simulink model "mpc_tgt_calc"  (R2022b)
settings: Solver=FixedStepDiscrete  StartTime=0.0  StopTime=2600  FixedStep=0.1  RelTol=1e-3
undefined symbols (not defined in the file): accl, alpha, alpha2, ang, beta, cnt_delay_accl_ratio, cnt_delay_decel_ratio, delay_accl, delay_v, dist, dt, ff_duty_front, ff_duty_l, ff_duty_r, ff_duty_roll, ff_duty_rpm_l, ff_duty_rpm_r, ideal_point, img_ang, img_dist, kanayama_point, pivot_state, sla_param, slip, slip_point, state, trj_diff, v, vx, vy, w
libraries: simulink_extras x1
(part 1 of 2)
settings Model: Creator=nao12  LastModifiedBy=naoto
settings SolverCC: AlgebraicLoopSolver=TrustRegion
settings DataIOCC: SaveOutput=off  SignalLogging=off  DSMLogging=off  SaveTime=off  ReturnWorkspaceOutputs=off
settings OptimizationCC: StrengthReduction=on  PassReuseOutputArgsAs=Individual arguments  ZeroExternalMemoryAtStartup=off  ZeroInternalMemoryAtStartup=off  OptimizeBlockOrder=speed  OptimizationPriority=Speed  OptimizationCustomize=off  MultiThreadedLoops=on  EfficientTunableParamExpr=on
settings DebuggingCC: ParameterTunabilityLossMsg=error  UnconnectedInputMsg=warning  UnconnectedOutputMsg=warning  UnconnectedLineMsg=warning  SFMachineParentedDataDiag=warning  ArithmeticOperatorsInVariantConditions=warning
settings ModelReferenceCC: EnableRefExpFcnMdlSchedulingChecks=on
settings SFSimCC: SimCustomHeaderCode="#include \"bus.h\""  SimUserIncludeDirs=../include/  MATLABDynamicMemAlloc=off  CustomCodeUndefinedFunction=UseInterfaceOnly  SimTargetLang=C++
settings RTWCC: Description=Embedded Coder  SystemTargetFile=ert.tlc  GenCodeOnly=on  TemplateMakefile=ert_default_tmf  GenerateReport=on  RTWUseSimCustomCode=on  CustomHeaderCode="#include \"bus.h\""  CustomInclude=../include/  Toolchain=GNU gcc/g++ | gmake (64-bit Linux)  IncludeHyperlinkInReport=on  LaunchReport=on  TargetLang=C++  GenerateTraceInfo=on  GenerateTraceReport=on  GenerateTraceReportSl=on  GenerateTraceReportSf=on  GenerateTraceReportEml=on  GenerateCodeMetricsReport=on  DLArmComputeVersion=19.05
settings CodeAppCC: GenerateComments=off  IgnoreCustomStorageClasses=off  OperatorAnnotations=on  SimulinkDataObjDesc=on  SFDataObjDesc=on  SimulinkBlockComments=off
settings ERTTargetCC: TargetLangStandard=C++11 (ISO)  GenerateSampleERTMain=on  SupportAbsoluteTime=off  CodeInterfacePackaging=C++ class  SupportComplex=off  ParenthesesLevel=Minimum  RootIOFormat=Structure reference  ERTCustomFileTemplate=example_file_process.tlc

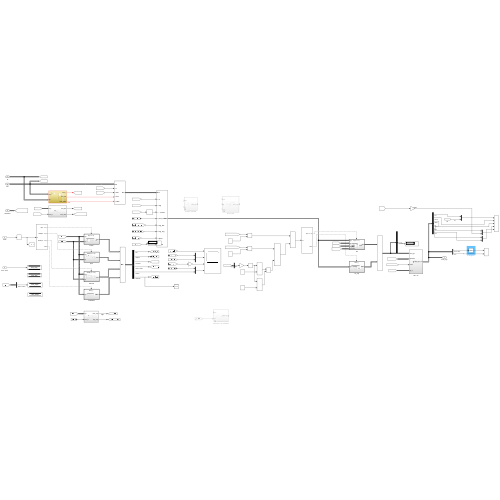
[thumbnail: Simulink's stored preview of the top-level diagram]
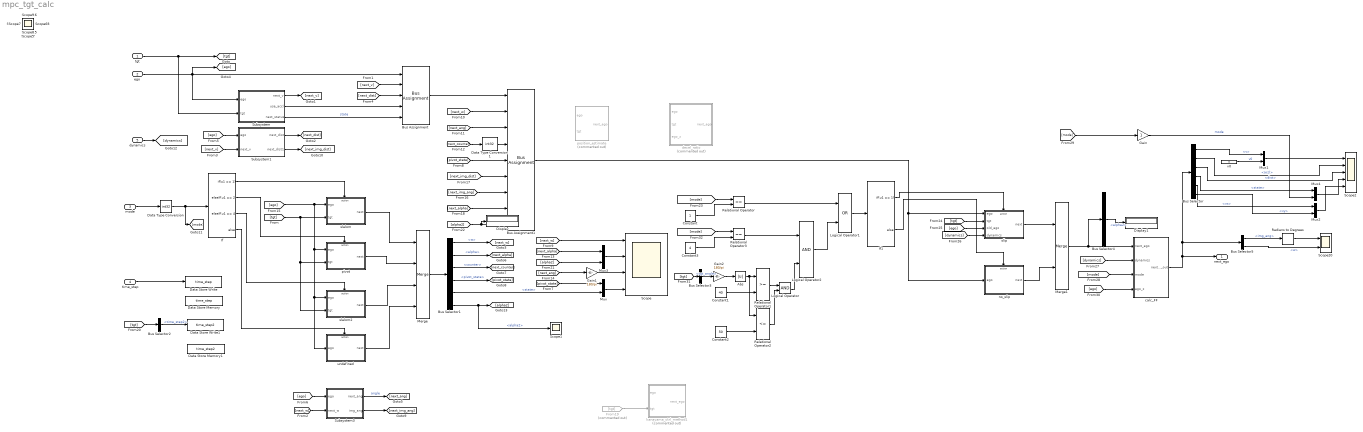
== system mpc_tgt_calc ==
  tgt : Inport  OutDataTypeStr=Bus: t_tgt  BusOutputAsStruct=on
  ego : Inport  Port=2  OutDataTypeStr=Bus: t_ego  BusOutputAsStruct=on
  mode : Inport  Port=3  OutDataTypeStr=int32
  time_step : Inport  Port=4  OutDataTypeStr=int32
  dynamics : Inport  Port=5  OutDataTypeStr=Bus: t_dynamics  BusOutputAsStruct=on
  Abs : Abs  SaturateOnIntegerOverflow=off
  Bus Assignment : BusAssignment  AssignedSignals=v,dist,accl,state
  Bus Assignment1 : BusAssignment  AssignedSignals=w,ang,sla_param.counter,pivot_state,img_dist,img_ang,alpha,alpha2
  Bus Selector : BusSelector  OutputSignals=v,accl,dist,state,slip.vx,slip.vy
  Bus Selector1 : BusSelector  OutputSignals=w,alpha,sla_param.counter,pivot_state,sla_param.state,alpha2
  Bus Selector2 : BusSelector  OutputSignals=time_step2
  Bus Selector3 : BusSelector  OutputSignals=tgt_angle
  Bus Selector4 : BusSelector  OutputSignals=alpha2
  Bus Selector5 : BusSelector  OutputSignals=img_ang,w
  Constant : Constant  OutDataTypeStr=int32
  Constant1 : Constant  Value=40  OutDataTypeStr=int32
  Constant2 : Constant  Value=50  OutDataTypeStr=int32
  Constant3 : Constant  Value=4  OutDataTypeStr=int32
  Data Store Memory : DataStoreMemory  DataStoreName=time_step  ReadBeforeWriteMsg=warning  WriteAfterWriteMsg=warning  WriteAfterReadMsg=warning  ShowAdditionalParam=off
  Data Store Memory1 : DataStoreMemory  DataStoreName=time_step2  ReadBeforeWriteMsg=warning  WriteAfterWriteMsg=warning  WriteAfterReadMsg=warning  ShowAdditionalParam=off
  Data Store Write : DataStoreWrite  DataStoreName=time_step  IndexOptions=Index vector (dialog)  Indices=1  OutputSizes=1
  Data Store Write1 : DataStoreWrite  DataStoreName=time_step2  IndexOptions=Index vector (dialog)  Indices=1  OutputSizes=1
  Data Type Conversion : DataTypeConversion  OutDataTypeStr=int32  SaturateOnIntegerOverflow=off  RndMeth=Floor
  Data Type Conversion1 : DataTypeConversion  OutDataTypeStr=int32  SaturateOnIntegerOverflow=off  RndMeth=Floor
  Display : Display
  Display1 : Display
  From19 : From  Commented=on  GotoTag=tgt
  Gain : Gain  OutDataTypeStr=int32
  Gain1 : Gain  Gain=180/pi
  Gain2 : Gain  Gain=180/pi
  If : If  IfExpression=u1 == 1  ElseIfExpressions=u1 == 2, u1 == 4
  If1 : If  IfExpression=u1 == 1
  Logical Operator : Logic  AllPortsSameDT=off  OutDataTypeStr=boolean
  Logical Operator1 : Logic  Operator=OR  AllPortsSameDT=off  OutDataTypeStr=boolean
  Logical Operator2 : Logic  AllPortsSameDT=off  OutDataTypeStr=boolean
  Merge : Merge  Inputs=4
  Merge1 : Merge
  Mux{,1..4} (5 alike) : Mux  Inputs=2
  Radians to Degrees : simulink_extras/Transformations/Radians to Degrees
  Relational Operator : RelationalOperator  Operator===  OutDataTypeStr=boolean  RndMeth=Simplest  InputSameDT=off
  Relational Operator1 : RelationalOperator  OutDataTypeStr=boolean  RndMeth=Simplest  InputSameDT=off
  Relational Operator2 : RelationalOperator  Operator=<=  OutDataTypeStr=boolean  RndMeth=Simplest  InputSameDT=off
  Relational Operator3 : RelationalOperator  Operator===  OutDataTypeStr=boolean  RndMeth=Simplest  InputSameDT=off
  Scope : Scope  NumInputPorts=4
  Scope{1,3..19} (18 alike) : Scope
  Scope2 : Scope  NumInputPorts=5
  Scope20 : Scope  NumInputPorts=2
  Subsystem : Subsystem
  Subsystem1 : Subsystem
  Subsystem3 : Subsystem
  calc_FF : Subsystem
  decel_ratio : Subsystem  Commented=on
  kanayama_ctrl_method1 : Subsystem  Commented=on
  no_slip : Subsystem  TreatAsAtomicUnit=on
  pivot : Subsystem  TreatAsAtomicUnit=on
  position_estimate : Subsystem  Commented=on
  slalom : Subsystem  TreatAsAtomicUnit=on
  slalom2 : Subsystem  TreatAsAtomicUnit=on
  slip : Subsystem  TreatAsAtomicUnit=on
  undefined : Subsystem  TreatAsAtomicUnit=on
  v0 : Constant  Value=0  OutDataTypeStr=single
  next_ego : Outport  OutDataTypeStr=Bus: t_ego
  wires:
  mode/1 -> Data Type Conversion/1
  tgt/1 -> [tgt], Subsystem/2(tgt)
  ego/1 -> Subsystem/1(ego), Bus Assignment/1, [ego]
  Data Type Conversion/1 -> [mode], If/1
  If/1 -> slalom/Action
  [tgt] -> slalom2/2(tgt), pivot/2(tgt), slalom/2(tgt)
  Bus Assignment/1 -> Bus Assignment1/1
  [next_v] -> Bus Assignment/2
  [next_dist] -> Bus Assignment/3
  Subsystem/1(next_v) -> [next_v]
  [next_v] -> Subsystem1/2(next_v)
  Subsystem1/1(next_dist) -> [next_dist]
  Subsystem/2(use_accl) -> Bus Assignment/4
  Subsystem/3(next_status) -> Bus Assignment/5  "state"
  [next_w] -> Subsystem3/2(next_w)
  [ego] -> Subsystem1/1(ego)
  [ego] -> Subsystem3/1(ego)
  Subsystem3/1(next_ang) -> [next_ang]  "angle"
  Bus Selector/4 -> Mux4/1  "<state>"
  Bus Selector/3 -> Scope2/3  "<dist>"
  [next_w] -> Bus Assignment1/2
  [next_ang] -> Bus Assignment1/3
  [next_counter] -> Data Type Conversion1/1
  Data Type Conversion1/1 -> Bus Assignment1/4
  [next_w] -> Scope/1
  [next_ang] -> Gain1/1
  If/2 -> pivot/Action
  [ego] -> slalom2/1(ego), undefined/1(ego), pivot/1(ego), slalom/1(ego)
  If/4 -> undefined/Action
  Merge/1 -> Bus Selector1/1
  Bus Selector1/1 -> [next_w]  "<w>"
  Bus Selector1/2 -> [next_alpha]  "<alpha>"
  Bus Selector1/3 -> [next_counter]  "<counter>"
  slalom/1(next) -> Merge/1
  pivot/1(next) -> Merge/2
  undefined/1(next) -> Merge/4
  Bus Selector1/4 -> [pivot_state]  "<pivot_state>"
  [pivot_state] -> Bus Assignment1/5
  Mux/1 -> Scope/4
  [pivot_state] -> Mux/1
  Bus Selector1/5 -> Mux/2  "<state>"
  Subsystem3/2(img_ang) -> [next_img_ang]
  [next_img_ang] -> Bus Assignment1/7
  Subsystem1/2(next_dist1) -> [next_img_dist]
  [next_img_dist] -> Bus Assignment1/6
  [next_alpha] -> Bus Assignment1/8
  From19/1 -> kanayama_ctrl_method1/2(tgt)
  time_step/1 -> Data Store Write/1
  slalom2/1(next) -> Merge/3
  If/3 -> slalom2/Action
  Bus Assignment1/1 -> no_slip/1(ego), slip/1(ego)
  If1/1 -> slip/Action
  slip/1(next) -> Merge1/1
  no_slip/1(next) -> Merge1/2
  If1/2 -> no_slip/Action
  Merge1/1 -> Bus Selector4/1, calc_FF/1(next_ego)
  [tgt] -> slip/2(tgt)
  [ego] -> slip/3(old_ego)
  Mux1/1 -> Scope2/1
  Bus Selector/1 -> Mux1/1  "<v>"
  v0/1 -> Mux1/2  "v0"
  [dynamics] -> calc_FF/2(dynamics)
  dynamics/1 -> [dynamics]
  [dynamics] -> slip/4(dynamics)
  Bus Selector2/1 -> Data Store Write1/1  "<time_step2>"
  [tgt] -> Bus Selector2/1
  Bus Selector1/6 -> Scope1/1, [alpha2]  "<alpha2>"
  Mux3/1 -> Scope/2
  [next_alpha] -> Mux3/1
  [alpha2] -> Mux3/2
  [alpha2] -> Display/1, Bus Assignment1/9
  calc_FF/1(next_ego_out) -> Bus Selector5/1, Bus Selector/1, next_ego/1
  [mode] -> calc_FF/3(mode)
  [mode] -> Gain/1
  Mux4/1 -> Scope2/4
  Gain/1 -> Mux4/2  "mode"
  Bus Selector/2 -> Scope2/2  "<accl>"
  Bus Selector/5 -> Mux2/1  "<vx>"
  Bus Selector/6 -> Mux2/2  "<vy>"
  Mux2/1 -> Scope2/5
  [ego] -> calc_FF/4(ego_z)
  Gain1/1 -> Scope/3
  [tgt] -> Bus Selector3/1
  Gain2/1 -> Abs/1
  [mode] -> Relational Operator/1
  Bus Selector3/1 -> Gain2/1  "<tgt_angle>"
  Relational Operator/1 -> Logical Operator1/1
  Constant/1 -> Relational Operator/2
  Abs/1 -> Relational Operator2/1, Relational Operator1/1
  Constant1/1 -> Relational Operator1/2
  Constant2/1 -> Relational Operator2/2
  Relational Operator1/1 -> Logical Operator/1
  Relational Operator2/1 -> Logical Operator/2
  Logical Operator1/1 -> If1/1
  [mode] -> Relational Operator3/1
  Relational Operator3/1 -> Logical Operator2/1
  Constant3/1 -> Relational Operator3/2
  Logical Operator/1 -> Logical Operator2/2
  Logical Operator2/1 -> Logical Operator1/2
  Bus Selector4/1 -> Display1/1  "<alpha2>"
  Bus Selector5/1 -> Radians to Degrees/1  "<img_ang>"
  Bus Selector5/2 -> Scope20/2  "<w>"
  Radians to Degrees/1 -> Scope20/1

== system mpc_tgt_calc/Subsystem ==
  ego : Inport
  tgt : Inport  Port=2
  Bus Selector2 : BusSelector  OutputSignals=v_max
  If : If  IfExpression=u1 >= 0
  Merge : Merge
  Merge1 : Merge
  Merge2 : Merge
  straight_ahead : Subsystem  TreatAsAtomicUnit=on
  straight_back : Subsystem  TreatAsAtomicUnit=on
  next_v : Outport
  use_accl : Outport  Port=2
  next_status : Outport  Port=3
  wires:
  tgt/1 -> [tgt], Bus Selector2/1
  Bus Selector2/1 -> If/1  "<v_max>"
  If/1 -> straight_ahead/Action
  ego/1 -> [ego]
  [ego] -> straight_ahead/1(ego)
  [tgt] -> straight_ahead/2(tgt)
  [ego] -> straight_back/1(ego)
  [tgt] -> straight_back/2(tgt)
  If/2 -> straight_back/Action
  straight_ahead/1(next_v) -> Merge/1
  straight_ahead/2(use_accl) -> Merge1/1
  straight_ahead/3(next_status) -> Merge2/1
  straight_back/1(next_v) -> Merge/2
  straight_back/2(use_accl) -> Merge1/2
  straight_back/3(next_status) -> Merge2/2
  Merge/1 -> next_v/1
  Merge1/1 -> use_accl/1
  Merge2/1 -> next_status/1

== system mpc_tgt_calc/Subsystem1 ==
  ego : Inport
  next_v : Inport  Port=2
  Add1 : Sum
  Add2 : Sum
  Bus Selector : BusSelector  OutputSignals=dist,img_dist
  Data Store Read : DataStoreRead  DataStoreName=time_step  IndexOptions=Index vector (dialog)  Indices=1  OutputSizes=1
  Data Type Conversion1 : DataTypeConversion  OutDataTypeStr=single  SaturateOnIntegerOverflow=off  RndMeth=Floor
  Data Type Conversion2 : DataTypeConversion  OutDataTypeStr=single  SaturateOnIntegerOverflow=off  RndMeth=Floor
  Data Type Conversion3 : DataTypeConversion  OutDataTypeStr=single  SaturateOnIntegerOverflow=off  RndMeth=Floor
  Gain1 : Gain  Gain=dt
  Product : Product
  next_dist : Outport
  next_dist1 : Outport  Port=2
  wires:
  ego/1 -> Bus Selector/1
  Bus Selector/1 -> Add1/1  "<dist>"
  Add1/1 -> Data Type Conversion1/1
  Data Type Conversion1/1 -> next_dist/1
  Add2/1 -> Data Type Conversion2/1
  Gain1/1 -> Add2/2, Add1/2
  Data Type Conversion2/1 -> next_dist1/1
  Bus Selector/2 -> Add2/1  "<img_dist>"
  Product/1 -> Gain1/1
  next_v/1 -> Product/1
  Data Store Read/1 -> Data Type Conversion3/1
  Data Type Conversion3/1 -> Product/2

== system mpc_tgt_calc/Subsystem3 ==
  ego : Inport
  next_w : Inport  Port=2
  Add1 : Sum
  Add2 : Sum
  Bus Selector : BusSelector  OutputSignals=ang,img_ang
  Data Store Read : DataStoreRead  DataStoreName=time_step  IndexOptions=Index vector (dialog)  Indices=1  OutputSizes=1
  Data Type Conversion1 : DataTypeConversion  OutDataTypeStr=single  SaturateOnIntegerOverflow=off  RndMeth=Floor
  Data Type Conversion2 : DataTypeConversion  OutDataTypeStr=single  SaturateOnIntegerOverflow=off  RndMeth=Floor
  Data Type Conversion3 : DataTypeConversion  OutDataTypeStr=single  SaturateOnIntegerOverflow=off  RndMeth=Floor
  Gain1 : Gain  Gain=dt
  Product : Product
  next_ang : Outport
  img_ang : Outport  Port=2
  wires:
  ego/1 -> Bus Selector/1
  Add1/1 -> Data Type Conversion1/1
  Bus Selector/1 -> Add1/1  "<ang>"
  Data Type Conversion1/1 -> next_ang/1
  Bus Selector/2 -> Add2/1  "<img_ang>"
  Data Type Conversion2/1 -> img_ang/1
  Add2/1 -> Data Type Conversion2/1
  Gain1/1 -> Add1/2, Add2/2
  Data Store Read/1 -> Data Type Conversion3/1
  Product/1 -> Gain1/1
  next_w/1 -> Product/1
  Data Type Conversion3/1 -> Product/2

== system mpc_tgt_calc/calc_FF ==
  next_ego : Inport
  dynamics : Inport  Port=2
  mode : Inport  Port=3
  ego_z : Inport  Port=4
  Add : Sum  Inputs=+-+
  Add1 : Sum  Inputs=+++
  Bus Assignment : BusAssignment  AssignedSignals=ff_duty_front,ff_duty_l,ff_duty_r,ff_duty_roll,ff_duty_rpm_r,ff_duty_rpm_l
  Mux : Mux  Inputs=2
  Mux1 : Mux  Inputs=2
  Scope : Scope  NumInputPorts=4
  Scope1 : Scope
  Subsystem : Subsystem
  calc_FF_Front : Subsystem
  calc_FF_Roll : Subsystem
  calc_counter_volt : Subsystem
  validation : Subsystem
  next_ego_out : Outport
  wires:
  next_ego/1 -> validation/1(next_ego)
  Bus Assignment/1 -> next_ego_out/1
  dynamics/1 -> calc_FF_Front/2(dynamics), calc_FF_Roll/2(dynamics), calc_counter_volt/2(dynamics)
  calc_counter_volt/1(left) -> [rpm_l_volt], Mux/1, Add/3  "rpm_l_volt"
  calc_counter_volt/2(right) -> Add1/3, [rpm_r_volt], Mux/2  "rpm_r_volt"
  Mux/1 -> Scope/4
  calc_FF_Front/1(front_volt) -> Subsystem/2(front_volt)
  calc_FF_Roll/1(roll_volt) -> [roll_volt], Scope1/1, Add1/2, Add/2, Scope/3
  Add1/1 -> Mux1/2, Bus Assignment/4  "FF_Right"
  Mux1/1 -> Scope/1
  Add/1 -> Mux1/1, Bus Assignment/3  "FF_Left"
  mode/1 -> Subsystem/3(mode)
  Subsystem/1(ff_front) -> Scope/2, Add1/1, Add/1, Bus Assignment/2
  validation/1(next_ego_out) -> calc_FF_Front/1(next_ego), calc_FF_Roll/1(next_ego), calc_counter_volt/1(next_ego), Subsystem/1(next_ego), Bus Assignment/1
  ego_z/1 -> validation/2(ego_z)
  [roll_volt] -> Bus Assignment/5
  [rpm_r_volt] -> Bus Assignment/6
  [rpm_l_volt] -> Bus Assignment/7

== system mpc_tgt_calc/decel_ratio ==
  ego : Inport
  tgt : Inport  Port=2
  ego_z : Inport  Port=3
  Bus Assignment : BusAssignment  AssignedSignals=delay_v,delay_accl,cnt_delay_accl_ratio,cnt_delay_decel_ratio
  Bus Selector : BusSelector  OutputSignals=accl
  Bus Selector1 : BusSelector  OutputSignals=v
  Data Store Read : DataStoreRead  DataStoreName=time_step  IndexOptions=Index vector (dialog)  Indices=1  OutputSizes=1
  Gain : Gain  Gain=dt
  If : If  ElseIfExpressions=u1 < 0
  If Action Subsystem : Subsystem  TreatAsAtomicUnit=on
  If Action Subsystem1 : Subsystem  TreatAsAtomicUnit=on
  If Action Subsystem2 : Subsystem  TreatAsAtomicUnit=on
  Merge : Merge  Inputs=3
  Merge1 : Merge  Inputs=3
  Merge2 : Merge  Inputs=3
  Product : Product
  next_ego : Outport
  wires:
  Bus Assignment/1 -> next_ego/1
  If/1 -> If Action Subsystem/Action
  ego/1 -> [ego], Bus Selector/1, Bus Assignment/1
  [ego] -> If Action Subsystem/1(ego)
  Bus Selector/1 -> If/1  "<accl>"
  tgt/1 -> If Action Subsystem/2(tgt), If Action Subsystem1/2(tgt)
  If/2 -> If Action Subsystem1/Action
  If/3 -> If Action Subsystem2/Action
  [ego] -> If Action Subsystem1/1(ego)
  If Action Subsystem/1(ff_accl) -> Merge/1
  If Action Subsystem1/1(ff_accl) -> Merge/2
  If Action Subsystem2/1(ff_accl) -> Merge/3
  If Action Subsystem/2(cnt_delay_accl_ratio) -> Merge1/1
  If Action Subsystem1/2(cnt_delay_accl_ratio) -> Merge1/2
  If Action Subsystem2/2(cnt_delay_accl_ratio) -> Merge1/3
  If Action Subsystem/3(cnt_delay_decel_ratio) -> Merge2/1
  If Action Subsystem1/3(cnt_delay_decel_ratio) -> Merge2/2
  If Action Subsystem2/3(cnt_delay_decel_ratio) -> Merge2/3
  Merge/1 -> Bus Assignment/3
  Merge1/1 -> Bus Assignment/4
  Merge2/1 -> Bus Assignment/5
  [ego] -> If Action Subsystem2/1(ego)
  ego_z/1 -> Bus Selector1/1
  Data Store Read/1 -> Product/1
  Gain/1 -> Product/2
  Bus Selector1/1 -> Gain/1  "<v>"
  Product/1 -> Bus Assignment/2

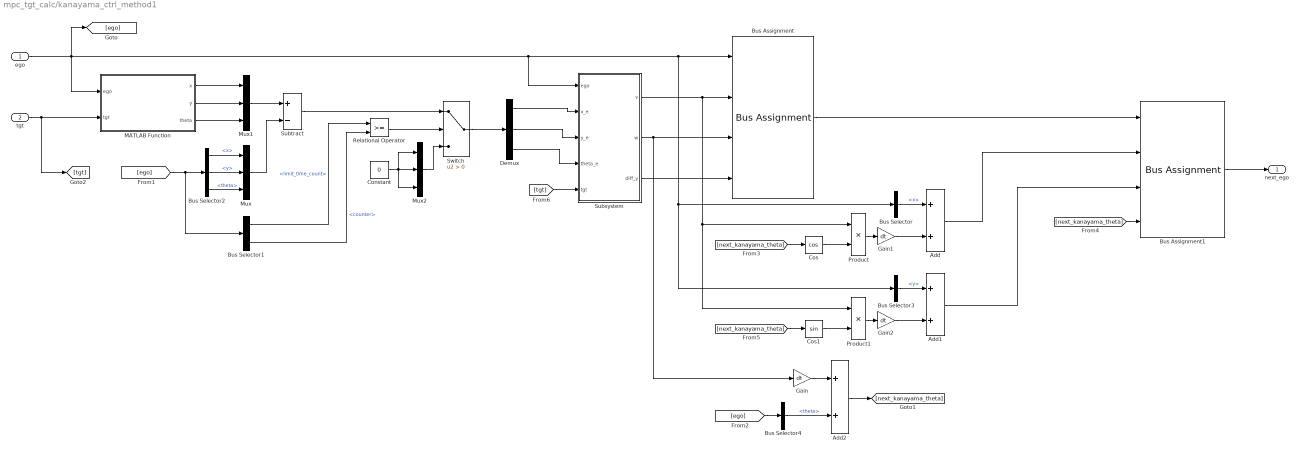
== system mpc_tgt_calc/kanayama_ctrl_method1 ==
  ego : Inport
  tgt : Inport  Port=2
  Add : Sum
  Add1 : Sum
  Add2 : Sum
  Bus Assignment : BusAssignment  AssignedSignals=kanayama_point.v,kanayama_point.w,kanayama_point.y
  Bus Assignment1 : BusAssignment  AssignedSignals=kanayama_point.x,kanayama_point.y,kanayama_point.theta
  Bus Selector : BusSelector  OutputSignals=kanayama_point.x
  Bus Selector1 : BusSelector  OutputSignals=sla_param.limit_time_count,sla_param.counter
  Bus Selector2 : BusSelector  OutputSignals=slip_point.x,slip_point.y,slip_point.theta
  Bus Selector3 : BusSelector  OutputSignals=kanayama_point.y
  Bus Selector4 : BusSelector  OutputSignals=kanayama_point.theta
  Constant : Constant  Value=0  OutDataTypeStr=single
  Cos : Trigonometry  Operator=cos
  Cos1 : Trigonometry
  Demux : Demux  Outputs=3
  Gain : Gain  Gain=dt
  Gain1 : Gain  Gain=dt
  Gain2 : Gain  Gain=dt
  MATLAB Function : MATLAB Function  TreatAsAtomicUnit=on
  Mux : Mux  Inputs=3
  Mux1 : Mux  Inputs=3
  Mux2 : Mux  Inputs=3
  Product : Product
  Product1 : Product
  Relational Operator : RelationalOperator  OutDataTypeStr=boolean  RndMeth=Simplest  InputSameDT=off
  Subsystem : Subsystem
  Subtract : Sum  Inputs=+-
  Switch : Switch  Criteria=u2 > Threshold  SaturateOnIntegerOverflow=off  InputSameDT=off
  next_ego : Outport
  wires:
  tgt/1 -> [tgt], MATLAB Function/2(tgt)
  Bus Selector2/1 -> Mux/1  "<x>"
  Bus Selector2/2 -> Mux/2  "<y>"
  Bus Selector2/3 -> Mux/3  "<theta>"
  MATLAB Function/1(x) -> Mux1/1
  MATLAB Function/2(y) -> Mux1/2
  MATLAB Function/3(theta) -> Mux1/3
  Mux1/1 -> Subtract/1
  Mux/1 -> Subtract/2
  Switch/1 -> Demux/1
  Bus Selector1/1 -> Relational Operator/1  "<limit_time_count>"
  Bus Selector1/2 -> Relational Operator/2  "<counter>"
  Relational Operator/1 -> Switch/2
  Subtract/1 -> Switch/1
  Mux2/1 -> Switch/3
  Constant/1 -> Mux2/1, Mux2/2, Mux2/3
  Bus Assignment/1 -> Bus Assignment1/1
  Demux/1 -> Subsystem/2(x_e)
  Demux/2 -> Subsystem/3(y_e)
  Demux/3 -> Subsystem/4(theta_e)
  Subsystem/2(w) -> Gain/1, Bus Assignment/3
  Product/1 -> Gain1/1
  Bus Selector/1 -> Add/1  "<x>"
  Add/1 -> Bus Assignment1/2
  Add1/1 -> Bus Assignment1/3
  Cos/1 -> Product/2
  Subsystem/1(v) -> Product/1, Product1/1, Bus Assignment/2
  [next_kanayama_theta] -> Cos/1
  Gain1/1 -> Add/2
  Cos1/1 -> Product1/2
  Gain2/1 -> Add1/2
  ego/1 -> MATLAB Function/1(ego), [ego], Subsystem/1(ego), Bus Selector3/1, Bus Selector/1, Bus Assignment/1
  Product1/1 -> Gain2/1
  Bus Assignment1/1 -> next_ego/1
  [ego] -> Bus Selector1/1, Bus Selector2/1
  [ego] -> Bus Selector4/1
  Gain/1 -> Add2/1
  Bus Selector4/1 -> Add2/2  "<theta>"
  Add2/1 -> [next_kanayama_theta]
  Bus Selector3/1 -> Add1/1  "<y>"
  [next_kanayama_theta] -> Bus Assignment1/4
  [next_kanayama_theta] -> Cos1/1
  [tgt] -> Subsystem/5(tgt)
  Subsystem/3(diff_y) -> Bus Assignment/4

== system mpc_tgt_calc/no_slip ==
  ego : Inport
  Action Port : ActionPort  ActionPortLabel=else
  Bus Assignment : BusAssignment  AssignedSignals=beta,vx,vy,v
  Bus Assignment1 : BusAssignment  AssignedSignals=slip
  Bus Selector : BusSelector  OutputSignals=slip,v
  Constant : Constant  Value=0  OutDataTypeStr=single
  Gain : Gain  Gain=0.001
  Gain1 : Gain  Gain=0.001
  next : Outport
  wires:
  Bus Assignment1/1 -> next/1
  Bus Selector/1 -> Bus Assignment/1  "<slip>"
  ego/1 -> Bus Selector/1, Bus Assignment1/1
  Bus Assignment/1 -> Bus Assignment1/2
  Constant/1 -> Bus Assignment/4, Bus Assignment/2
  Bus Selector/2 -> Gain/1, Gain1/1  "<v>"
  Gain/1 -> Bus Assignment/5
  Gain1/1 -> Bus Assignment/3

== system mpc_tgt_calc/pivot ==
  ego : Inport
  tgt : Inport  Port=2
  Action Port : ActionPort  ActionPortLabel=elseif(u1 == 2)
  Abs : Abs  SaturateOnIntegerOverflow=off
  Abs1 : Abs  SaturateOnIntegerOverflow=off
  Add : Sum
  Bus Assignment : BusAssignment  AssignedSignals=w,alpha,alpha2,pivot_state
  Bus Assignment1 : BusAssignment  AssignedSignals=w,alpha,alpha2,pivot_state
  Bus Selector : BusSelector  OutputSignals=w
  Bus Selector1 : BusSelector  OutputSignals=ang
  Bus Selector2 : BusSelector  OutputSignals=tgt_angle
  Constant : Constant  Value=0  OutDataTypeStr=single
  Constant1 : Constant  Value=3  OutDataTypeStr=int32
  Data Store Read : DataStoreRead  DataStoreName=time_step  IndexOptions=Index vector (dialog)  Indices=1  OutputSizes=1
  Data Type Conversion1 : DataTypeConversion  OutDataTypeStr=single  SaturateOnIntegerOverflow=off  RndMeth=Floor
  Data Type Conversion2 : DataTypeConversion  OutDataTypeStr=single  SaturateOnIntegerOverflow=off  RndMeth=Floor
  Data Type Conversion3 : DataTypeConversion  OutDataTypeStr=single  SaturateOnIntegerOverflow=off  RndMeth=Floor
  Gain : Gain  Gain=dt
  Product : Product
  Relational Operator1 : RelationalOperator  Operator=<  OutDataTypeStr=boolean  RndMeth=Simplest  InputSameDT=off
  Subsystem : Subsystem
  Switch2 : Switch  Criteria=u2 > Threshold  SaturateOnIntegerOverflow=off  InputSameDT=off
  next : Outport
  wires:
  ego/1 -> Subsystem/1(ego), Bus Selector/1, Bus Assignment/1, [ego]
  Subsystem/1(next_alpha) -> Data Type Conversion1/1, Gain/1
  Bus Selector/1 -> Add/1  "<w>"
  Add/1 -> Data Type Conversion2/1
  Data Type Conversion2/1 -> Bus Assignment/2
  tgt/1 -> [tgt], Subsystem/2(tgt)
  Data Type Conversion1/1 -> Bus Assignment/4, Bus Assignment/3
  Subsystem/2(state_out) -> Bus Assignment/5
  Bus Assignment/1 -> Bus Assignment1/1, Switch2/1
  Relational Operator1/1 -> Switch2/2
  Bus Selector2/1 -> Abs1/1  "<tgt_angle>"
  Abs/1 -> Relational Operator1/1
  [ego] -> Bus Selector1/1
  [tgt] -> Bus Selector2/1
  Bus Selector1/1 -> Abs/1  "<ang>"
  Abs1/1 -> Relational Operator1/2
  Switch2/1 -> next/1
  Constant/1 -> Bus Assignment1/4, Bus Assignment1/3, Bus Assignment1/2
  Constant1/1 -> Bus Assignment1/5
  Bus Assignment1/1 -> Switch2/3
  Data Store Read/1 -> Data Type Conversion3/1
  Gain/1 -> Product/1
  Product/1 -> Add/2
  Data Type Conversion3/1 -> Product/2

== system mpc_tgt_calc/position_estimate ==
  ego : Inport
  tgt : Inport  Port=2
  Add : Sum
  Add1 : Sum
  Bus Assignment : BusAssignment  AssignedSignals=ideal_point.x,ideal_point.y,ideal_point.theta
  Bus Assignment1 : BusAssignment  AssignedSignals=trj_diff.x,trj_diff.y,trj_diff.theta
  Bus Selector : BusSelector  OutputSignals=ideal_point.x,v,img_ang
  Bus Selector1 : BusSelector  OutputSignals=ideal_point.y,v,img_ang
  Bus Selector2 : BusSelector  OutputSignals=ideal_point.theta
  Bus Selector3 : BusSelector  OutputSignals=ideal_point.x,ideal_point.y
  Bus Selector4 : BusSelector  OutputSignals=slip_point.x,slip_point.y
  Bus Selector5 : BusSelector  OutputSignals=img_ang,slip_point.theta
  Cos : Trigonometry  Operator=cos
  Cos1 : Trigonometry
  Data Store Read1 : DataStoreRead  DataStoreName=time_step  IndexOptions=Index vector (dialog)  Indices=1  OutputSizes=1
  Gain1 : Gain  Gain=dt
  Gain2 : Gain  Gain=dt
  Gain5 : Gain
  Gain6 : Gain
  Mux : Mux  Inputs=2
  Mux1 : Mux  Inputs=2
  Product{,1..3} (4 alike) : Product
  Scope : Scope  NumInputPorts=2
  Subtract : Sum  Inputs=+-
  Subtract1 : Sum  Inputs=+-
  Subtract2 : Sum  Inputs=+-
  slipped_position_estimate : Subsystem
  next_ego : Outport
  wires:
  ego/1 -> slipped_position_estimate/1(ego), Bus Selector1/1, Bus Selector2/1, Bus Selector/1
  Bus Selector/1 -> Add/1  "<x>"
  Bus Selector/2 -> Product/1  "<v>"
  Bus Selector/3 -> Cos/1  "<img_ang>"
  Cos/1 -> Product/2
  Product/1 -> Gain1/1
  Bus Selector1/2 -> Product1/1  "<v>"
  Bus Selector1/1 -> Add1/1  "<y>"
  Product1/1 -> Gain2/1
  Bus Selector1/3 -> Cos1/1  "<img_ang>"
  Cos1/1 -> Product1/2
  Bus Selector2/1 -> Bus Assignment/4  "<theta>"
  Add1/1 -> Bus Assignment/3
  Add/1 -> Bus Assignment/2
  Bus Selector3/1 -> Subtract/1  "<x>"
  Bus Selector3/2 -> Subtract1/1  "<y>"
  slipped_position_estimate/1(next_ego) -> Bus Assignment/1
  Bus Selector4/1 -> Subtract/2  "<x>"
  Bus Selector4/2 -> Subtract1/2  "<y>"
  Subtract/1 -> Bus Assignment1/2, Mux1/1  "slip_diff_x"
  Subtract1/1 -> Mux1/2, Bus Assignment1/3  "slip_diff_y"
  Bus Assignment/1 -> Bus Selector5/1, Bus Selector3/1, Bus Assignment1/1, Bus Selector4/1
  Bus Selector5/2 -> Gain6/1  "<theta>"
  Gain6/1 -> Mux/2, Subtract2/2  "slipped_angle"
  Gain5/1 -> Mux/1, Subtract2/1  "ideal_angle"
  Bus Selector5/1 -> Gain5/1  "<img_ang>"
  Mux/1 -> Scope/2
  Mux1/1 -> Scope/1
  Bus Assignment1/1 -> next_ego/1
  Subtract2/1 -> Bus Assignment1/4  "slip_diff_theta"
  tgt/1 -> slipped_position_estimate/2(tgt)
  Product2/1 -> Add/2
  Gain1/1 -> Product2/1
  Product3/1 -> Add1/2
  Data Store Read1/1 -> Product3/1, Product2/2
  Gain2/1 -> Product3/2

== system mpc_tgt_calc/slalom ==
  ego : Inport
  tgt : Inport  Port=2
  Action Port : ActionPort  ActionPortLabel=if(u1 == 1)
  Bus Assignment : BusAssignment  AssignedSignals=w,alpha,sla_param.counter,alpha2
  Data Type Conversion : DataTypeConversion  OutDataTypeStr=int32  SaturateOnIntegerOverflow=off  RndMeth=Floor
  Data Type Conversion1 : DataTypeConversion  OutDataTypeStr=single  SaturateOnIntegerOverflow=off  RndMeth=Floor
  Data Type Conversion2 : DataTypeConversion  OutDataTypeStr=single  SaturateOnIntegerOverflow=off  RndMeth=Floor
  Data Type Conversion3 : DataTypeConversion  OutDataTypeStr=single  SaturateOnIntegerOverflow=off  RndMeth=Floor
  Subsystem2 : Subsystem
  next : Outport
  wires:
  ego/1 -> Subsystem2/1(ego), Bus Assignment/1
  tgt/1 -> Subsystem2/2(tgt)
  Bus Assignment/1 -> next/1
  Subsystem2/1(next_w) -> Data Type Conversion1/1
  Subsystem2/2(next_alpha) -> Data Type Conversion2/1
  Subsystem2/3(next_count) -> Data Type Conversion/1
  Data Type Conversion/1 -> Bus Assignment/4
  Data Type Conversion1/1 -> Bus Assignment/2
  Data Type Conversion2/1 -> Bus Assignment/3
  Data Type Conversion3/1 -> Bus Assignment/5
  Subsystem2/4(next_alpha2) -> Data Type Conversion3/1

== system mpc_tgt_calc/slalom2 ==
  ego : Inport
  tgt : Inport  Port=2
  Action Port : ActionPort  ActionPortLabel=elseif( u1 == 4)
  Abs : Abs  SaturateOnIntegerOverflow=off
  Abs1 : Abs  SaturateOnIntegerOverflow=off
  Add : Sum
  Bus Assignment : BusAssignment  AssignedSignals=w,alpha,pivot_state
  Bus Assignment1 : BusAssignment  AssignedSignals=w,alpha,alpha2,pivot_state
  Bus Selector : BusSelector  OutputSignals=w
  Bus Selector1 : BusSelector  OutputSignals=img_ang
  Bus Selector2 : BusSelector  OutputSignals=tgt_angle
  Bus Selector3 : BusSelector  OutputSignals=w
  Constant : Constant  Value=0  OutDataTypeStr=single
  Constant1 : Constant  Value=3  OutDataTypeStr=int32
  Data Store Read : DataStoreRead  DataStoreName=time_step  IndexOptions=Index vector (dialog)  Indices=1  OutputSizes=1
  Data Store Read1 : DataStoreRead  DataStoreName=time_step  IndexOptions=Index vector (dialog)  Indices=1  OutputSizes=1
  Data Type Conversion{1..4} (4 alike) : DataTypeConversion  OutDataTypeStr=single  SaturateOnIntegerOverflow=off  RndMeth=Floor
  Divide : Product  Inputs=*/
  Gain : Gain  Gain=dt
  Gain1 : Gain  Gain=dt
  Product : Product
  Relational Operator1 : RelationalOperator  Operator=<  OutDataTypeStr=boolean  RndMeth=Simplest  InputSameDT=off
  Scope : Scope
  Subsystem : Subsystem
  Subtract : Sum  Inputs=+-
  Switch2 : Switch  Criteria=u2 > Threshold  SaturateOnIntegerOverflow=off  InputSameDT=off
  next : Outport
  wires:
  Subsystem/1(next_alpha) -> Data Type Conversion1/1, Gain/1
  Bus Selector/1 -> Add/1  "<w>"
  Add/1 -> Data Type Conversion2/1
  Data Type Conversion2/1 -> Bus Assignment/2
  Data Type Conversion1/1 -> Bus Assignment/3
  Subsystem/2(state_out) -> Bus Assignment/4
  Bus Assignment/1 -> Bus Assignment1/1, Switch2/1
  Relational Operator1/1 -> Switch2/2
  Bus Selector2/1 -> Abs1/1  "<tgt_angle>"
  Abs/1 -> Relational Operator1/1
  ego/1 -> Bus Selector3/1, Subsystem/1(ego), Bus Selector/1, Bus Selector1/1, Bus Assignment/1
  tgt/1 -> Bus Selector2/1, Subsystem/2(tgt)
  Bus Selector1/1 -> Abs/1  "<img_ang>"
  Abs1/1 -> Relational Operator1/2
  Switch2/1 -> next/1
  Constant1/1 -> Bus Assignment1/5
  Bus Assignment1/1 -> Switch2/3
  Data Store Read/1 -> Data Type Conversion3/1
  Gain/1 -> Product/1
  Product/1 -> Add/2
  Constant/1 -> Subtract/1, Bus Assignment1/4, Bus Assignment1/3, Bus Assignment1/2
  Bus Selector3/1 -> Subtract/2  "<w>"
  Subtract/1 -> Divide/1
  Data Store Read1/1 -> Data Type Conversion4/1
  Gain1/1 -> Divide/2
  Data Type Conversion3/1 -> Product/2
  Data Type Conversion4/1 -> Gain1/1

== system mpc_tgt_calc/slip ==
  ego : Inport
  tgt : Inport  Port=2
  old_ego : Inport  Port=3
  dynamics : Inport  Port=4
  Action Port : ActionPort  ActionPortLabel=if(u1 == 1)
  Bus Assignment1 : BusAssignment  AssignedSignals=slip,v,accl
  Bus Selector3 : BusSelector  OutputSignals=v
  Subsystem : Subsystem
  next : Outport
  wires:
  ego/1 -> Subsystem/1(next_ego), Bus Assignment1/1
  Bus Assignment1/1 -> next/1
  old_ego/1 -> Bus Selector3/1
  Subsystem/1(slip_param) -> Bus Assignment1/2
  tgt/1 -> Subsystem/2(tgt)
  Bus Selector3/1 -> Subsystem/3(old_v)  "<v>"
  Subsystem/2(v) -> Bus Assignment1/3
  Subsystem/3(accl) -> Bus Assignment1/4
  dynamics/1 -> Subsystem/4(dynamics)

== system mpc_tgt_calc/undefined ==
  ego : Inport
  Action Port : ActionPort  ActionPortLabel=else
  Bus Assignment1 : BusAssignment  AssignedSignals=w,alpha,alpha2
  Bus Selector3 : BusSelector  OutputSignals=w
  Constant : Constant  Value=0  OutDataTypeStr=single
  Data Store Read : DataStoreRead  DataStoreName=time_step  IndexOptions=Index vector (dialog)  Indices=1  OutputSizes=1
  Data Type Conversion1 : DataTypeConversion  OutDataTypeStr=single  SaturateOnIntegerOverflow=off  RndMeth=Floor
  Data Type Conversion2 : DataTypeConversion  OutDataTypeStr=single  SaturateOnIntegerOverflow=off  RndMeth=Floor
  Divide : Product  Inputs=*/
  Gain : Gain  Gain=dt
  Subtract : Sum  Inputs=+-
  next : Outport
  wires:
  ego/1 -> Bus Selector3/1, Bus Assignment1/1
  Gain/1 -> Divide/2
  Bus Selector3/1 -> Subtract/2  "<w>"
  Subtract/1 -> Divide/1
  Constant/1 -> Subtract/1, Bus Assignment1/2
  Divide/1 -> Bus Assignment1/4, Bus Assignment1/3
  Bus Assignment1/1 -> next/1
  Data Store Read/1 -> Data Type Conversion1/1
  Data Type Conversion1/1 -> Gain/1

== system mpc_tgt_calc/Subsystem/straight_ahead ==
  ego : Inport
  tgt : Inport  Port=2
  Action Port : ActionPort  ActionPortLabel=if(u1 >= 0)
  Add : Sum
  Bus Selector : BusSelector  OutputSignals=v
  Bus Selector1 : BusSelector  OutputSignals=v_max
  Constant : Constant  Value=0  OutDataTypeStr=single
  Data Store Read : DataStoreRead  DataStoreName=time_step  IndexOptions=Index vector (dialog)  Indices=1  OutputSizes=1
  Data Type Conversion1 : DataTypeConversion  OutDataTypeStr=single  SaturateOnIntegerOverflow=off  RndMeth=Floor
  Data Type Conversion2 : DataTypeConversion  OutDataTypeStr=single  SaturateOnIntegerOverflow=off  RndMeth=Floor
  Gain : Gain  Gain=dt
  Max : MinMax  Function=max  Inputs=2
  Min : MinMax  Inputs=2
  Product : Product
  Subsystem : Subsystem
  next_v : Outport
  use_accl : Outport  Port=2
  next_status : Outport  Port=3
  wires:
  Max/1 -> next_v/1
  Subsystem/1(use_accl) -> use_accl/1, Gain/1
  Constant/1 -> Max/2
  Bus Selector/1 -> Add/1  "<v>"
  ego/1 -> Subsystem/1(ego), Bus Selector/1
  tgt/1 -> Subsystem/2(tgt), Bus Selector1/1
  Data Type Conversion2/1 -> Min/2
  Min/1 -> Max/1  "velocity"
  Bus Selector1/1 -> Min/1  "<v_max>"
  Subsystem/2(next_state) -> next_status/1
  Add/1 -> Data Type Conversion2/1
  Data Store Read/1 -> Data Type Conversion1/1
  Product/1 -> Add/2
  Gain/1 -> Product/2
  Data Type Conversion1/1 -> Product/1

== system mpc_tgt_calc/Subsystem/straight_back ==
  ego : Inport
  tgt : Inport  Port=2
  Action Port : ActionPort  ActionPortLabel=else
  Add : Sum
  Bus Selector : BusSelector  OutputSignals=v
  Bus Selector1 : BusSelector  OutputSignals=v_max
  Constant : Constant  Value=0  OutDataTypeStr=single
  Data Store Read : DataStoreRead  DataStoreName=time_step  IndexOptions=Index vector (dialog)  Indices=1  OutputSizes=1
  Data Type Conversion1 : DataTypeConversion  OutDataTypeStr=single  SaturateOnIntegerOverflow=off  RndMeth=Floor
  Data Type Conversion2 : DataTypeConversion  OutDataTypeStr=single  SaturateOnIntegerOverflow=off  RndMeth=Floor
  Gain : Gain  Gain=dt
  Max : MinMax  Inputs=2
  Min : MinMax  Function=max  Inputs=2
  Product : Product
  Subsystem : Subsystem
  next_v : Outport
  use_accl : Outport  Port=2
  next_status : Outport  Port=3
  wires:
  Max/1 -> next_v/1
  Subsystem/1(use_accl) -> use_accl/1, Gain/1
  Constant/1 -> Max/2
  Bus Selector/1 -> Add/1  "<v>"
  ego/1 -> Subsystem/1(ego), Bus Selector/1
  tgt/1 -> Subsystem/2(tgt), Bus Selector1/1
  Data Type Conversion2/1 -> Min/2
  Min/1 -> Max/1  "velocity"
  Bus Selector1/1 -> Min/1  "<v_max>"
  Subsystem/2(next_state) -> next_status/1
  Add/1 -> Data Type Conversion2/1
  Data Store Read/1 -> Data Type Conversion1/1
  Product/1 -> Add/2
  Gain/1 -> Product/2
  Data Type Conversion1/1 -> Product/1

== system mpc_tgt_calc/calc_FF/Subsystem ==
  next_ego : Inport
  front_volt : Inport  Port=2
  mode : Inport  Port=3
  Bus Selector : BusSelector  OutputSignals=state
  If : If  NumInputs=2  IfExpression=(u2==0 | u2==3 ) & (u1==0)
  If Action Subsystem : Subsystem  TreatAsAtomicUnit=on
  If Action Subsystem1 : Subsystem  TreatAsAtomicUnit=on
  Merge : Merge
  ff_front : Outport
  wires:
  next_ego/1 -> If Action Subsystem/2(next_ego), Bus Selector/1
  Bus Selector/1 -> If/1  "<state>"
  mode/1 -> If/2
  If/1 -> If Action Subsystem/Action
  If/2 -> If Action Subsystem1/Action
  front_volt/1 -> If Action Subsystem1/1(front_volt), If Action Subsystem/1(front_volt)
  If Action Subsystem/1(Out1) -> Merge/1
  If Action Subsystem1/1(Out1) -> Merge/2
  Merge/1 -> ff_front/1

== system mpc_tgt_calc/calc_FF/calc_FF_Front ==
  next_ego : Inport
  dynamics : Inport  Port=2
  Bus Selector : BusSelector  OutputSignals=accl
  Bus Selector1 : BusSelector  OutputSignals=mass,tire,resist
  Bus Selector2 : BusSelector  OutputSignals=gear_ratio,km
  Divide : Product  Inputs=*/
  Gain1 : Gain  Gain=0.001
  Gain4 : Gain  Gain=0.001
  Product : Product  Inputs=4
  Product1 : Product
  front_volt : Outport
  wires:
  Bus Selector1/1 -> Product/2  "<mass>"
  dynamics/1 -> Bus Selector2/1, Bus Selector1/1
  next_ego/1 -> Bus Selector/1
  Bus Selector/1 -> Gain4/1  "<accl>"
  Gain4/1 -> Product/1
  Bus Selector1/2 -> Gain1/1  "<tire>"
  Bus Selector1/3 -> Product/4  "<resist>"
  Gain1/1 -> Product/3
  Bus Selector2/2 -> Product1/2  "<km>"
  Bus Selector2/1 -> Product1/1  "<gear_ratio>"
  Product/1 -> Divide/1
  Product1/1 -> Divide/2
  Divide/1 -> front_volt/1

== system mpc_tgt_calc/calc_FF/calc_FF_Roll ==
  next_ego : Inport
  dynamics : Inport  Port=2
  Bus Selector : BusSelector  OutputSignals=alpha2
  Bus Selector1 : BusSelector  OutputSignals=lm,tire,resist
  Bus Selector2 : BusSelector  OutputSignals=gear_ratio,km,tread
  Display{,1..5} (6 alike) : Display
  Divide : Product  Inputs=*/
  Divide1 : Product  Inputs=*/
  Gain1 : Gain  Gain=0.001
  Gain2 : Gain  Gain=0.001
  Product : Product  Inputs=4
  Product1 : Product
  Scope : Scope  NumInputPorts=2
  Scope2 : Scope
  roll_volt : Outport
  wires:
  Bus Selector1/3 -> Product/4, Display5/1  "<resist>"
  Bus Selector/1 -> Display3/1, Product/1  "<alpha2>"
  Bus Selector1/2 -> Gain1/1  "<tire>"
  next_ego/1 -> Bus Selector/1
  Bus Selector1/1 -> Display4/1, Product/2  "<lm>"
  dynamics/1 -> Bus Selector2/1, Bus Selector1/1
  Product1/1 -> Display2/1, Divide/2
  Gain1/1 -> Product/3
  Divide/1 -> Scope/1, Display/1, Divide1/1
  Product/1 -> Display1/1, Divide/1
  Bus Selector2/1 -> Product1/1  "<gear_ratio>"
  Bus Selector2/2 -> Product1/2  "<km>"
  Bus Selector2/3 -> Gain2/1  "<tread>"
  Gain2/1 -> Divide1/2, Scope2/1
  Divide1/1 -> roll_volt/1

== system mpc_tgt_calc/calc_FF/calc_counter_volt ==
  next_ego : Inport
  dynamics : Inport  Port=2
  Add : Sum  Inputs=+-
  Add1 : Sum
  Bus Selector : BusSelector  OutputSignals=v,w
  Bus Selector1 : BusSelector  OutputSignals=tread
  Bus Selector2 : BusSelector  OutputSignals=ke,tire
  Divide : Product  Inputs=*/
  Divide1 : Product  Inputs=*/
  Gain : Gain  Gain=0.5
  Gain1 : Gain  Gain=0.5
  Gain2 : Gain  Gain=30/pi
  Gain3 : Gain  Gain=30/pi
  Gain4 : Gain  Gain=0.001
  Gain5 : Gain  Gain=0.001
  Gain6 : Gain  Gain=0.001
  Product : Product
  Product1 : Product
  Product2 : Product
  left : Outport
  right : Outport  Port=2
  wires:
  next_ego/1 -> Bus Selector/1
  dynamics/1 -> Bus Selector2/1, Bus Selector1/1
  Bus Selector/1 -> Gain4/1  "<v>"
  Bus Selector/2 -> Product/1  "<w>"
  Bus Selector1/1 -> Gain5/1  "<tread>"
  Gain/1 -> Product/2
  Product/1 -> Add1/2, Add/2
  Add/1 -> Product1/1
  Add1/1 -> Product2/1
  Bus Selector2/1 -> [ke]  "<ke>"
  Bus Selector2/2 -> Gain6/1  "<tire>"
  Gain1/1 -> [tire_2]
  [ke] -> Product1/2
  Product1/1 -> Gain2/1
  [tire_2] -> Divide/2
  [tire_2] -> Divide1/2
  Gain2/1 -> Divide/1
  Product2/1 -> Gain3/1
  Gain3/1 -> Divide1/1
  [ke] -> Product2/2
  Divide/1 -> left/1
  Divide1/1 -> right/1
  Gain4/1 -> Add1/1, Add/1
  Gain5/1 -> Gain/1
  Gain6/1 -> Gain1/1

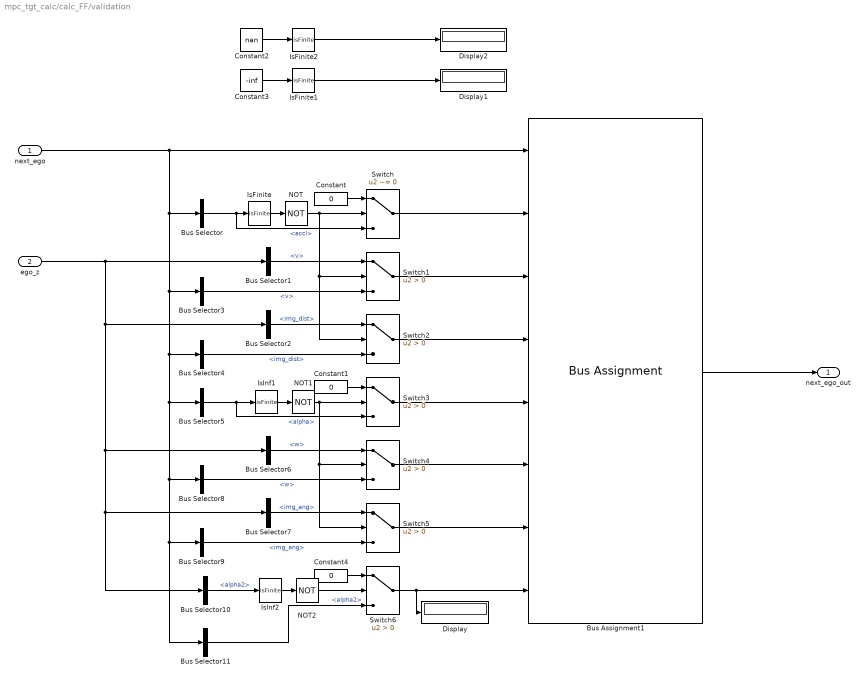
== system mpc_tgt_calc/calc_FF/validation ==
  next_ego : Inport
  ego_z : Inport  Port=2
  Bus Assignment1 : BusAssignment  AssignedSignals=accl,v,img_dist,alpha,w,img_ang,alpha2
  Bus Selector : BusSelector  OutputSignals=accl
  Bus Selector1 : BusSelector  OutputSignals=v
  Bus Selector10 : BusSelector  OutputSignals=alpha2
  Bus Selector11 : BusSelector  OutputSignals=alpha2
  Bus Selector2 : BusSelector  OutputSignals=img_dist
  Bus Selector3 : BusSelector  OutputSignals=v
  Bus Selector4 : BusSelector  OutputSignals=img_dist
  Bus Selector5 : BusSelector  OutputSignals=alpha
  Bus Selector6 : BusSelector  OutputSignals=w
  Bus Selector7 : BusSelector  OutputSignals=img_ang
  Bus Selector8 : BusSelector  OutputSignals=w
  Bus Selector9 : BusSelector  OutputSignals=img_ang
  Constant : Constant  Value=0  OutDataTypeStr=single
  Constant1 : Constant  Value=0  OutDataTypeStr=single
  Constant2 : Constant  Value=nan
  Constant3 : Constant  Value=-inf
  Constant4 : Constant  Value=0  OutDataTypeStr=single
  Display : Display
  Display1 : Display
  Display2 : Display
  IsFinite : RelationalOperator  Operator=isFinite  OutDataTypeStr=boolean  RndMeth=Simplest  InputSameDT=off
  IsFinite1 : RelationalOperator  Operator=isFinite  OutDataTypeStr=boolean  RndMeth=Simplest  InputSameDT=off
  IsFinite2 : RelationalOperator  Operator=isFinite  OutDataTypeStr=boolean  RndMeth=Simplest  InputSameDT=off
  IsInf1 : RelationalOperator  Operator=isFinite  OutDataTypeStr=boolean  RndMeth=Simplest  InputSameDT=off
  IsInf2 : RelationalOperator  Operator=isFinite  OutDataTypeStr=boolean  RndMeth=Simplest  InputSameDT=off
  NOT : Logic  Operator=NOT  IconShape=distinctive  AllPortsSameDT=off  OutDataTypeStr=boolean
  NOT1 : Logic  Operator=NOT  IconShape=distinctive  AllPortsSameDT=off  OutDataTypeStr=boolean
  NOT2 : Logic  Operator=NOT  IconShape=distinctive  AllPortsSameDT=off  OutDataTypeStr=boolean
  Switch : Switch  Criteria=u2 ~= 0  SaturateOnIntegerOverflow=off  InputSameDT=off
  Switch{1..6} (6 alike) : Switch  Criteria=u2 > Threshold  SaturateOnIntegerOverflow=off  InputSameDT=off
  next_ego_out : Outport
  wires:
  Bus Selector/1 -> IsFinite/1, Switch/3  "<accl>"
  Switch/1 -> Bus Assignment1/2
  Constant/1 -> Switch/1
  Bus Assignment1/1 -> next_ego_out/1
  Bus Selector1/1 -> Switch1/1  "<v>"
  Switch1/1 -> Bus Assignment1/3
  IsFinite/1 -> NOT/1
  Bus Selector2/1 -> Switch2/1  "<img_dist>"
  Switch2/1 -> Bus Assignment1/4
  Bus Selector3/1 -> Switch1/3  "<v>"
  Bus Selector4/1 -> Switch2/3  "<img_dist>"
  Bus Selector6/1 -> Switch4/1  "<w>"
  Switch3/1 -> Bus Assignment1/5
  Constant1/1 -> Switch3/1
  Switch4/1 -> Bus Assignment1/6
  Bus Selector8/1 -> Switch4/3  "<w>"
  Switch5/1 -> Bus Assignment1/7
  Bus Selector5/1 -> Switch3/3, IsInf1/1  "<alpha>"
  next_ego/1 -> Bus Selector11/1, Bus Selector9/1, Bus Selector8/1, Bus Selector5/1, Bus Selector4/1, Bus Selector3/1, Bus Selector/1, Bus Assignment1/1
  IsInf1/1 -> NOT1/1
  Bus Selector7/1 -> Switch5/1  "<img_ang>"
  Bus Selector9/1 -> Switch5/3  "<img_ang>"
  IsFinite1/1 -> Display1/1
  IsFinite2/1 -> Display2/1
  Constant2/1 -> IsFinite2/1
  Constant3/1 -> IsFinite1/1
  NOT/1 -> Switch2/2, Switch1/2, Switch/2
  NOT1/1 -> Switch5/2, Switch4/2, Switch3/2
  Switch6/1 -> Display/1, Bus Assignment1/8
  Bus Selector10/1 -> IsInf2/1  "<alpha2>"
  ego_z/1 -> Bus Selector6/1, Bus Selector10/1, Bus Selector7/1, Bus Selector2/1, Bus Selector1/1
  IsInf2/1 -> NOT2/1
  NOT2/1 -> Switch6/2
  Constant4/1 -> Switch6/1
  Bus Selector11/1 -> Switch6/3  "<alpha2>"

== system mpc_tgt_calc/decel_ratio/If Action Subsystem ==
  ego : Inport
  tgt : Inport  Port=2
  Action Port : ActionPort  ActionPortLabel=if(u1 > 0)
  Add : Sum
  Bus Selector : BusSelector  OutputSignals=cnt_delay_accl_ratio,cnt_delay_decel_ratio
  Bus Selector1 : BusSelector  OutputSignals=accl
  Bus Selector2 : BusSelector  OutputSignals=limit_accl_ratio_cnt
  Constant : Constant  OutDataTypeStr=single
  Constant1 : Constant  OutDataTypeStr=single
  Divide : Product  Inputs=*/
  Product : Product
  Saturation : Saturate  UpperLimit=1  LowerLimit=0
  Switch : Switch  Criteria=u2 ~= 0  SaturateOnIntegerOverflow=off  InputSameDT=off
  ff_accl : Outport
  cnt_delay_accl_ratio : Outport  Port=2
  cnt_delay_decel_ratio : Outport  Port=3
  wires:
  ego/1 -> Bus Selector1/1, Bus Selector/1
  Bus Selector/1 -> Add/1  "<cnt_delay_accl_ratio>"
  Constant/1 -> Add/2
  Bus Selector/2 -> cnt_delay_decel_ratio/1  "<cnt_delay_decel_ratio>"
  Add/1 -> cnt_delay_accl_ratio/1, Divide/1
  tgt/1 -> Bus Selector2/1
  Divide/1 -> Saturation/1
  Saturation/1 -> Product/2
  Product/1 -> ff_accl/1
  Bus Selector1/1 -> Product/1  "<accl>"
  Constant1/1 -> Switch/3
  Bus Selector2/1 -> Switch/2, Switch/1  "<limit_accl_ratio_cnt>"
  Switch/1 -> Divide/2

== system mpc_tgt_calc/decel_ratio/If Action Subsystem1 ==
  ego : Inport
  tgt : Inport  Port=2
  Action Port : ActionPort  ActionPortLabel=elseif(u1 < 0)
  Add : Sum
  Bus Selector : BusSelector  OutputSignals=cnt_delay_decel_ratio,cnt_delay_accl_ratio
  Bus Selector1 : BusSelector  OutputSignals=accl
  Bus Selector2 : BusSelector  OutputSignals=limit_decel_ratio_cnt
  Constant : Constant  OutDataTypeStr=single
  Constant1 : Constant  OutDataTypeStr=single
  Divide : Product  Inputs=*/
  Product : Product
  Saturation : Saturate  UpperLimit=1  LowerLimit=0
  Switch : Switch  Criteria=u2 ~= 0  SaturateOnIntegerOverflow=off  InputSameDT=off
  ff_accl : Outport
  cnt_delay_accl_ratio : Outport  Port=2
  cnt_delay_decel_ratio : Outport  Port=3
  wires:
  Product/1 -> ff_accl/1
  Bus Selector2/1 -> Switch/1, Switch/2  "<limit_decel_ratio_cnt>"
  Add/1 -> cnt_delay_decel_ratio/1, Divide/1
  Divide/1 -> Saturation/1
  Saturation/1 -> Product/2
  ego/1 -> Bus Selector/1, Bus Selector1/1
  Constant/1 -> Add/2
  Bus Selector1/1 -> Product/1  "<accl>"
  tgt/1 -> Bus Selector2/1
  Bus Selector/1 -> Add/1  "<cnt_delay_decel_ratio>"
  Bus Selector/2 -> cnt_delay_accl_ratio/1  "<cnt_delay_accl_ratio>"
  Switch/1 -> Divide/2
  Constant1/1 -> Switch/3

== system mpc_tgt_calc/decel_ratio/If Action Subsystem2 ==
  ego : Inport
  Action Port : ActionPort  ActionPortLabel=else
  Bus Selector : BusSelector  OutputSignals=accl,cnt_delay_accl_ratio,cnt_delay_decel_ratio
  ff_accl : Outport
  cnt_delay_accl_ratio : Outport  Port=2
  cnt_delay_decel_ratio : Outport  Port=3
  wires:
  ego/1 -> Bus Selector/1
  Bus Selector/1 -> ff_accl/1  "<accl>"
  Bus Selector/2 -> cnt_delay_accl_ratio/1  "<cnt_delay_accl_ratio>"
  Bus Selector/3 -> cnt_delay_decel_ratio/1  "<cnt_delay_decel_ratio>"

== system mpc_tgt_calc/kanayama_ctrl_method1/Subsystem ==
  ego : Inport
  x_e : Inport  Port=2
  y_e : Inport  Port=3
  theta_e : Inport  Port=4
  tgt : Inport  Port=5
  Add : Sum
  Add1 : Sum
  Bus Selector : BusSelector  OutputSignals=v,w
  Bus Selector1 : BusSelector  OutputSignals=kanayama_gain.k_x,kanayama_gain.k_y,kanayama_gain.k_theta
  Cos : Trigonometry  Operator=cos
  Data Type Conversion : DataTypeConversion  OutDataTypeStr=single  SaturateOnIntegerOverflow=off  RndMeth=Floor
  Data Type Conversion1 : DataTypeConversion  OutDataTypeStr=single  SaturateOnIntegerOverflow=off  RndMeth=Floor
  Product : Product
  Product1 : Product
  Product2 : Product
  Scope : Scope
  v : Outport
  w : Outport  Port=2
  diff_y : Outport  Port=3
  wires:
  ego/1 -> Bus Selector/1
  tgt/1 -> Bus Selector1/1
  Bus Selector1/1 -> [k_x]  "<k_x>"
  Bus Selector1/2 -> [k_y]  "<k_y>"
  Bus Selector1/3 -> [k_theta]  "<k_theta>"
  Bus Selector/1 -> [ideal_v]  "<v>"
  Bus Selector/2 -> [ideal_w]  "<w>"
  [ideal_v] -> Product/1
  Cos/1 -> Product/2
  Product/1 -> Add/1
  Product1/1 -> Add/2
  [k_x] -> Product1/1
  [ideal_w] -> Add1/1
  Add/1 -> Data Type Conversion/1
  Data Type Conversion/1 -> v/1
  theta_e/1 -> Scope/1, Cos/1
  Add1/1 -> Data Type Conversion1/1
  Data Type Conversion1/1 -> w/1
  x_e/1 -> Product1/2
  Product2/1 -> Add1/2
  y_e/1 -> diff_y/1, Product2/2
  [k_y] -> Product2/1

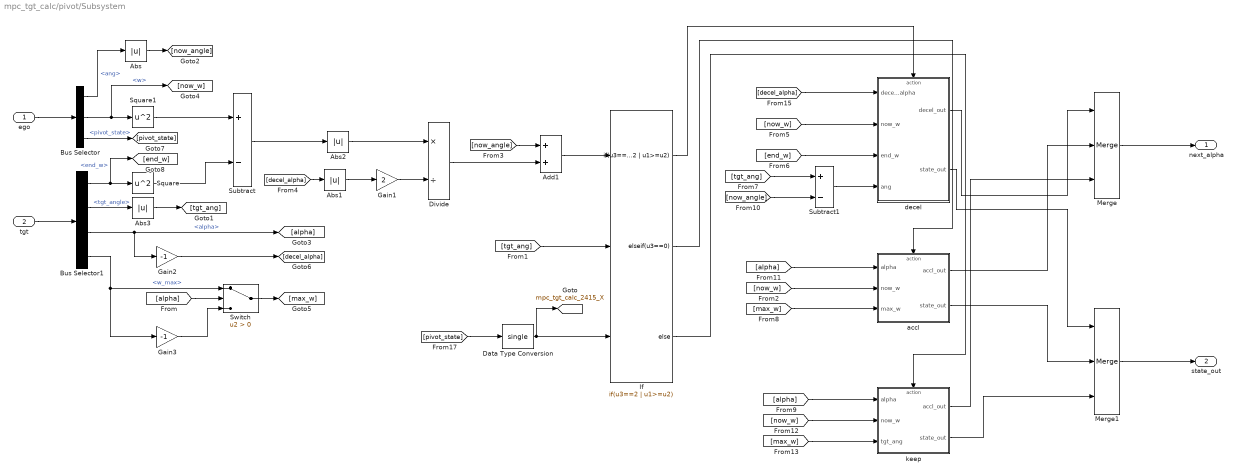
== system mpc_tgt_calc/pivot/Subsystem ==
  ego : Inport
  tgt : Inport  Port=2
  Abs{,1..3} (4 alike) : Abs  SaturateOnIntegerOverflow=off
  Add1 : Sum
  Bus Selector : BusSelector  OutputSignals=ang,w,pivot_state
  Bus Selector1 : BusSelector  OutputSignals=end_w,tgt_angle,alpha,w_max
  Data Type Conversion : DataTypeConversion  OutDataTypeStr=single  SaturateOnIntegerOverflow=off  RndMeth=Floor
  Divide : Product  Inputs=*/
  Gain1 : Gain  Gain=2
  Gain2 : Gain  Gain=-1
  Gain3 : Gain  Gain=-1
  If : If  NumInputs=3  IfExpression=u3==2 | u1>=u2  ElseIfExpressions=u3==0
  Merge : Merge  Inputs=3
  Merge1 : Merge  Inputs=3
  Square : Math  Operator=square
  Square1 : Math  Operator=square
  Subtract : Sum  Inputs=+-
  Subtract1 : Sum  Inputs=+-
  Switch : Switch  Criteria=u2 > Threshold  SaturateOnIntegerOverflow=off  InputSameDT=off
  accl : Subsystem  TreatAsAtomicUnit=on
  decel : Subsystem  TreatAsAtomicUnit=on
  keep : Subsystem  TreatAsAtomicUnit=on
  next_alpha : Outport
  state_out : Outport  Port=2
  tag scope: mpc_tgt_calc_2415_X=global
  wires:
  ego/1 -> Bus Selector/1
  Subtract/1 -> Abs2/1
  Divide/1 -> Add1/2
  [now_angle] -> Add1/1
  Abs1/1 -> Gain1/1
  Abs2/1 -> Divide/1
  [decel_alpha] -> Abs1/1
  Gain1/1 -> Divide/2
  tgt/1 -> Bus Selector1/1
  Bus Selector1/1 -> [end_w], Square/1  "<end_w>"
  Square/1 -> Subtract/2
  Square1/1 -> Subtract/1
  Bus Selector/3 -> [pivot_state]  "<pivot_state>"
  Bus Selector/2 -> [now_w], Square1/1  "<w>"
  Bus Selector/1 -> Abs/1  "<ang>"
  Bus Selector1/2 -> Abs3/1  "<tgt_angle>"
  Bus Selector1/3 -> Gain2/1, [alpha]  "<alpha>"
  Gain2/1 -> [decel_alpha]
  Switch/1 -> [max_w]
  [alpha] -> Switch/2
  Bus Selector1/4 -> Gain3/1, Switch/1  "<w_max>"
  Gain3/1 -> Switch/3
  [pivot_state] -> Data Type Conversion/1
  Data Type Conversion/1 -> If/3, [mpc_tgt_calc_2415_X]
  [tgt_ang] -> If/2
  Add1/1 -> If/1
  keep/2(state_out) -> Merge1/3
  decel/1(decel_out) -> Merge/1
  [max_w] -> keep/3(tgt_ang)
  accl/1(accl_out) -> Merge/2
  [now_w] -> keep/2(now_w)
  [decel_alpha] -> decel/1(decel_alpha)
  [now_w] -> decel/2(now_w)
  [now_angle] -> Subtract1/2
  [tgt_ang] -> Subtract1/1
  [now_w] -> accl/2(now_w)
  accl/2(state_out) -> Merge1/2
  If/2 -> accl/Action
  keep/1(accl_out) -> Merge/3
  [max_w] -> accl/3(max_w)
  [alpha] -> keep/1(alpha)
  If/3 -> keep/Action
  [end_w] -> decel/3(end_w)
  decel/2(state_out) -> Merge1/1
  Merge1/1 -> state_out/1
  Subtract1/1 -> decel/4(ang)
  If/1 -> decel/Action
  Merge/1 -> next_alpha/1
  [alpha] -> accl/1(alpha)
  Abs/1 -> [now_angle]
  Abs3/1 -> [tgt_ang]
